simulink model "Detection"  (R2014b)
settings: Solver=ode45  StartTime=0.0  StopTime=10.0  RelTol=1e-3
undefined symbols (not defined in the file): strel, template_detection
libraries: visionstatistics x1, visionmorphops x1, simulink x1
settings Model: Creator=Jackie  LastModifiedBy=Jackie

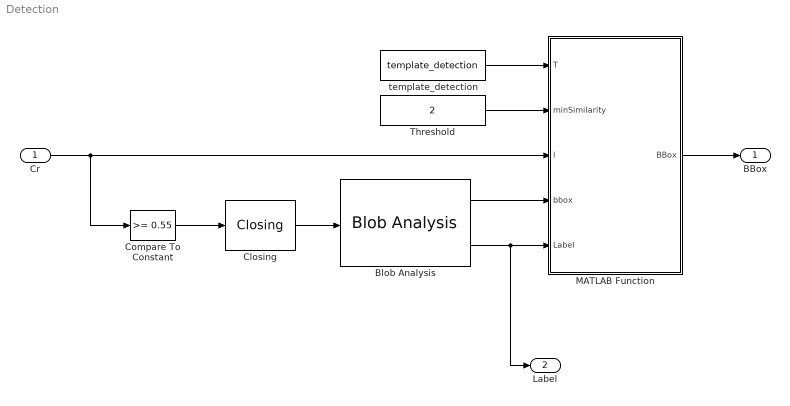
== system Detection ==
  Cr : Inport
  Blob Analysis : visionstatistics/Blob Analysis  Tag=vipblks_row_conv  area=off  centroid=off  bBox=on  majorAxis=off  minorAxis=off  angle=off  eccentricity=off  equivDiameterSq=off  extent=off  perimeter=off  maxBlobs=100000  warnIfNumBlobsExceeded=on  isCount=off  useMinArea=off  minArea=0  useMaxArea=off  maxArea=intmax('uint32')  excludeBorderBlob=off  outDT=single  isOutVarDim=on  isFill=on  fillValues=-1  conn=8  isLabel=on  outputMode=Binary point scaling  outputWordLength=32  outputFracLength=16  firstCoeffMode=Binary point scaling  firstCoeffWordLength=16  firstCoeffFracLength=14  secondCoeffMode=Binary point scaling  secondCoeffWordLength=32  secondCoeffFracLength=16  accumMode=Binary point scaling  accumWordLength=32  accumFracLength=0  prodOutputMode=Binary point scaling  prodOutputWordLength=32  prodOutputFracLength=16  roundingMode=Floor  overflowMode=off
  Closing : visionmorphops/Closing  nhoodsrc=Specify via dialog  strel=strel('line',5,45)
  Compare To Constant : simulink/Logic and Bit Operations/Compare To Constant  relop=>=  const=0.55  OutDataTypeStr=boolean
  MATLAB Function : MATLAB Function  TreatAsAtomicUnit=on
  Threshold : Constant  Value=2
  template_detection : Constant  Value=template_detection  OutDataTypeStr=single
  BBox : Outport
  Label : Outport  Port=2
  wires:
  Closing/1 -> Blob Analysis/1
  Compare To Constant/1 -> Closing/1
  Cr/1 -> MATLAB Function/3(I), Compare To Constant/1
  MATLAB Function/1(BBox) -> BBox/1
  Threshold/1 -> MATLAB Function/2(minSimilarity)
  Blob Analysis/2 -> MATLAB Function/5(Label), Label/1
  Blob Analysis/1 -> MATLAB Function/4(bbox)
  template_detection/1 -> MATLAB Function/1(T)

== matlab function Detection/MATLAB Function ==
  data: T input; BBox output; minSimilarity input; I input; bbox input; Label input
function BBox = Detection(T, minSimilarity, I, bbox, Label)
% This function finds the targets that are similar enough to any of the 
% templates. Similarity measure is calculated by correlation.
%
% Input:
%    T: 
%       Templates. Size is M-by-N-by-K, where M and N are the number of
%       rows and the number of columns in each template, respectively.
%       K is the number of templates.
%    minSimilarity: 
%       The minimum similarity a potential target and any of 
%       the templates must have in order for the blob to be considered as 
%       a valid target.
%    I: 
%       Intensity image under test.
%    bbox: 
%       Bounding boxes of the potential targets. Each column has the
%       format of [r, c, h, w] and corresponds to a potential target.
%    Label: 
%       Labeled image. Pixels from the same potential target have
%       the same label.
%
% Output:
%    BBox: 
%       Bounding boxes of the valid targets. 

numImgRows = single(size(Label, 2));
numImgCols = single(size(Label, 1));
numTmpRows = single(size(T, 1));
numTmpCols = single(size(T, 2));
numTemplates = single(size(T, 3));
numBBox = single(size(bbox, 1));
feature = single(zeros(numTmpRows, numTmpCols));
BBox = single(zeros(numBBox,4));


for idx = 1: numBBox
    bestSimilarity = single(0);
    
    if bbox(idx,4)>=numTmpRows && bbox(idx,3)>=numTmpCols
        % Step sizes for calculating features
        stepRows = floor(single(bbox(idx,4)) / numTmpRows);
        stepCols = floor(single(bbox(idx,3)) / numTmpCols);
        
        % Each side of the bounding box has been tried on three different
        % positions.
        startColList = single(zeros(1, 3));
        startColList(2) = bbox(idx,1);
        startColList(1) = max(1, startColList(2)-stepCols);
        startColList(3) = min(numImgCols, startColList(2)+stepCols);
        
        endColList = single(zeros(1, 3));
        endColList(2) = bbox(idx,1)+bbox(idx,3)-1;
        endColList(1) = max(1, endColList(2)-stepCols);
        endColList(3) = min(numImgCols, endColList(2)+stepCols);
        
        startRowList = single(zeros(1, 3));
        startRowList(2) = bbox(idx,2);
        startRowList(1) = max(1, startRowList(2)-stepRows);
        startRowList(3) = min(numImgRows, startRowList(2)+stepRows);
        
        endRowList = single(zeros(1, 3));
        endRowList(2) = bbox(idx,2)+bbox(idx,4)-1;
        endRowList(1) = max(1, endRowList(2)-stepRows);
        endRowList(3) = min(numImgRows, endRowList(2)+stepRows);
        
        % Try all possible positions for bouding box and find the best match
        for startCol = startColList
            for endCol = endColList
                ratioCols = (endCol - startCol) / numTmpCols;
                for startRow = startRowList
                    for endRow = endRowList
                        ratioRows = (endRow - startRow) / numTmpRows;
                        
                        % Calculate features
                        colSrcFlt = startCol;
                        for col = 1: numTmpCols
                            colSrc = floor(colSrcFlt);
                            rowSrcFlt = startRow;
                            for row = 1: numTmpRows
                                rowSrc = floor(rowSrcFlt);
                                feature(row, col) = I(rowSrc,colSrc);
                                rowSrcFlt = rowSrcFlt + ratioRows;
                            end
                            colSrcFlt = colSrcFlt + ratioCols;
                        end
                        
                        % Normalization
                        feature = feature - mean(feature(:));
                            
                        % Match with each of the templates
                        for iTmp = 1: numTemplates
                            similarity = single(0);
                            % Correlation
                            for col = 1: numTmpCols
                                for row = 1: numTmpRows
                                    similarity = similarity ...
                                        + T(row,col,iTmp)*feature(row,col);
                                end
                            end
                            if similarity > bestSimilarity
                                bestSimilarity = similarity;
                            end
                        end
                    end
                end
            end
        end
        
        % Output the valid targets
        if bestSimilarity>=minSimilarity
            BBox(idx,1) = bbox(idx,1);
            BBox(idx,2) = bbox(idx,2);
            BBox(idx,3) = bbox(idx,3);
            BBox(idx,4) = bbox(idx,4);
        end
    end
end
